simulink subsystem "Automotive_PowerTrain_AWDDifferential"  (R2024a)
settings: Solver=VariableStepAuto  StartTime=0.0  StopTime=10.0  RelTol=1e-3
libraries: autolibshareddiff x1
settings Model: Creator=USER  LastModifiedBy=USER

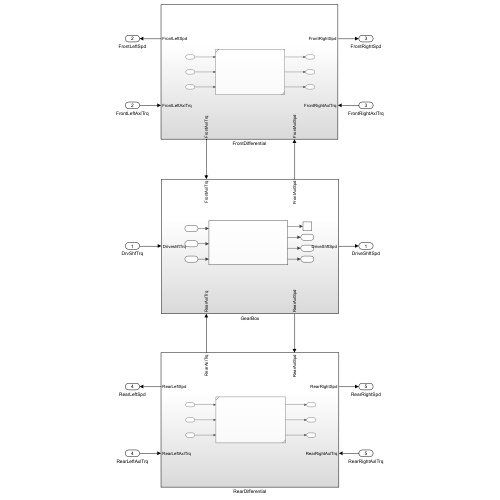
[thumbnail: Simulink's stored preview of the top-level diagram]
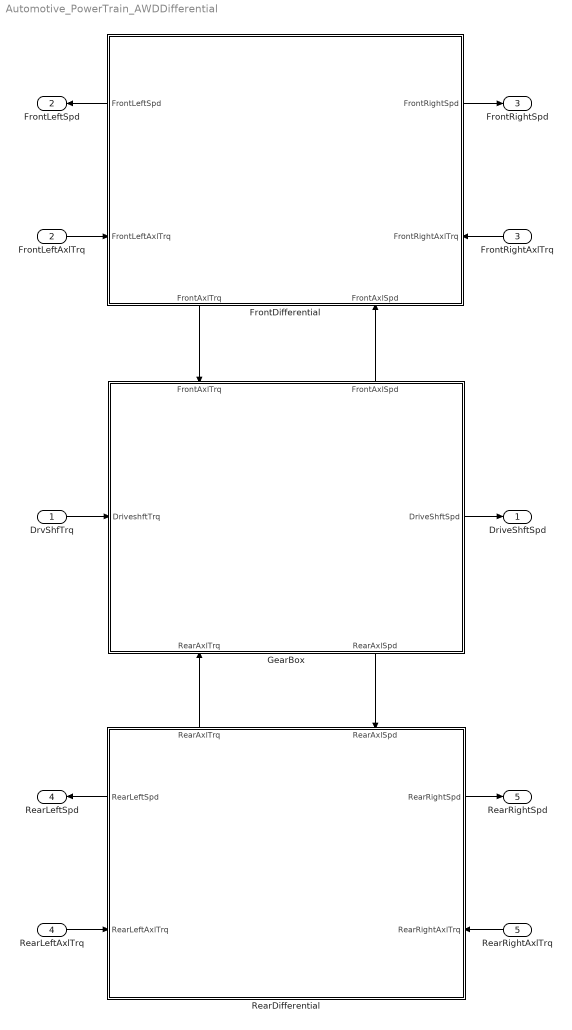
== system Automotive_PowerTrain_AWDDifferential ==
  DrvShfTrq : Inport
  FrontLeftAxlTrq : Inport  Port=2
  FrontRightAxlTrq : Inport  Port=3
  RearLeftAxlTrq : Inport  Port=4
  RearRightAxlTrq : Inport  Port=5
  FrontDifferential : Subsystem
      settings: PortSchema="{\"entries\":[{\"content\":{\"sides\":[{\"content\":{\"connectorIds\":[\"Out3\",\"In1\"]},\"type\":\"ConnectorPlacement.EquallySpacedRectSide\",\"uuid\":\"27f3256e-89ab-4368-8c78-2db926080991\"},{\"content\":{\"connectorIds\":[\"Out1\",\"In3\"],\"side\":\"RIGHT\"},\"type\":\"ConnectorPlacement.EquallySpacedRectSide\",\"uuid\":\"36e842ff-c4c6-4a20-acdc-cd70f8986d21\"},{\"content\":{\"side\":\"TOP\"},\"type\":\"ConnectorPlacement.EquallySpacedRectSide\",\"uuid\":\"2ccb2f9c-d9f3-4252-bb7a-d9380f21ab32\"},{\"content\":{\"connectorIds\":[\"Out2\",\"In2\"],\"side\":\"BOTTOM\"},\"type\":\"ConnectorPlacement.EquallySpacedRectSide\",\"uuid\":\"96e6a735-73c3-4e47-8511-c3716bbb9bc8\"}]},\"type\":\"ConnectorPlacement.EquallySpacedConnector\",\"uuid\":\"e81dde65-7a38-434f-9640-9946cbffd07c\"}],\"packageUris\":[\"http://schema.mathworks.com/mf0/Connector/R2020b\"],\"version\":\"1.0\"}"
  GearBox : Subsystem
      settings: PortSchema="{\"entries\":[{\"content\":{\"sides\":[{\"content\":{\"connectorIds\":[\"In1\"]},\"type\":\"ConnectorPlacement.EquallySpacedRectSide\",\"uuid\":\"27f3256e-89ab-4368-8c78-2db926080991\"},{\"content\":{\"connectorIds\":[\"Out1\"],\"side\":\"RIGHT\"},\"type\":\"ConnectorPlacement.EquallySpacedRectSide\",\"uuid\":\"36e842ff-c4c6-4a20-acdc-cd70f8986d21\"},{\"content\":{\"connectorIds\":[\"In2\",\"Out3\"],\"side\":\"TOP\"},\"type\":\"ConnectorPlacement.EquallySpacedRectSide\",\"uuid\":\"2ccb2f9c-d9f3-4252-bb7a-d9380f21ab32\"},{\"content\":{\"connectorIds\":[\"In3\",\"Out2\"],\"side\":\"BOTTOM\"},\"type\":\"ConnectorPlacement.EquallySpacedRectSide\",\"uuid\":\"f764fb99-6446-42c8-aaa9-dec82b0a64e1\"}]},\"type\":\"ConnectorPlacement.EquallySpacedConnector\",\"uuid\":\"e81dde65-7a38-434f-9640-9946cbffd07c\"}],\"packageUris\":[\"http://schema.mathworks.com/mf0/Connector/R2020b\"],\"version\":\"1.0\"}"
  RearDifferential : Subsystem
      settings: PortSchema="{\"entries\":[{\"content\":{\"sides\":[{\"content\":{\"connectorIds\":[\"Out3\",\"In1\"]},\"type\":\"ConnectorPlacement.EquallySpacedRectSide\",\"uuid\":\"27f3256e-89ab-4368-8c78-2db926080991\"},{\"content\":{\"connectorIds\":[\"Out1\",\"In3\"],\"side\":\"RIGHT\"},\"type\":\"ConnectorPlacement.EquallySpacedRectSide\",\"uuid\":\"36e842ff-c4c6-4a20-acdc-cd70f8986d21\"},{\"content\":{\"connectorIds\":[\"Out2\",\"In2\"],\"side\":\"TOP\"},\"type\":\"ConnectorPlacement.EquallySpacedRectSide\",\"uuid\":\"2ccb2f9c-d9f3-4252-bb7a-d9380f21ab32\"},{\"content\":{\"side\":\"BOTTOM\"},\"type\":\"ConnectorPlacement.EquallySpacedRectSide\",\"uuid\":\"96e6a735-73c3-4e47-8511-c3716bbb9bc8\"}]},\"type\":\"ConnectorPlacement.EquallySpacedConnector\",\"uuid\":\"e81dde65-7a38-434f-9640-9946cbffd07c\"}],\"packageUris\":[\"http://schema.mathworks.com/mf0/Connector/R2020b\"],\"version\":\"1.0\"}"
  DriveShftSpd : Outport
  FrontLeftSpd : Outport  Port=2
  FrontRightSpd : Outport  Port=3
  RearLeftSpd : Outport  Port=4
  RearRightSpd : Outport  Port=5
  wires:
  DrvShfTrq/1 -> GearBox/1(DriveshftTrq)
  GearBox/1(DriveShftSpd) -> DriveShftSpd/1
  FrontDifferential/2(FrontAxlTrq) -> GearBox/2(FrontAxlTrq)
  GearBox/3(FrontAxlSpd) -> FrontDifferential/2(FrontAxlSpd)
  RearDifferential/2(RearAxlTrq) -> GearBox/3(RearAxlTrq)
  GearBox/2(RearAxlSpd) -> RearDifferential/2(RearAxlSpd)
  FrontLeftAxlTrq/1 -> FrontDifferential/1(FrontLeftAxlTrq)
  FrontRightAxlTrq/1 -> FrontDifferential/3(FrontRightAxlTrq)
  RearLeftAxlTrq/1 -> RearDifferential/1(RearLeftAxlTrq)
  RearRightAxlTrq/1 -> RearDifferential/3(RearRightAxlTrq)
  FrontDifferential/3(FrontLeftSpd) -> FrontLeftSpd/1
  FrontDifferential/1(FrontRightSpd) -> FrontRightSpd/1
  RearDifferential/3(RearLeftSpd) -> RearLeftSpd/1
  RearDifferential/1(RearRightSpd) -> RearRightSpd/1

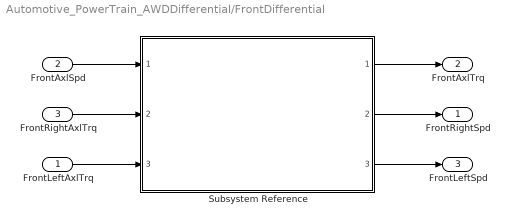
== system Automotive_PowerTrain_AWDDifferential/FrontDifferential ==
  FrontLeftAxlTrq : Inport
  FrontAxlSpd : Inport  Port=2
  FrontRightAxlTrq : Inport  Port=3
  Subsystem Reference : Subsystem  ReferencedSubsystem=Automotive_PowerTrain_OpenDifferential
  FrontRightSpd : Outport
  FrontAxlTrq : Outport  Port=2
  FrontLeftSpd : Outport  Port=3
  wires:
  FrontAxlSpd/1 -> Subsystem Reference/1
  FrontRightAxlTrq/1 -> Subsystem Reference/2
  FrontLeftAxlTrq/1 -> Subsystem Reference/3
  Subsystem Reference/1 -> FrontAxlTrq/1
  Subsystem Reference/3 -> FrontLeftSpd/1
  Subsystem Reference/2 -> FrontRightSpd/1

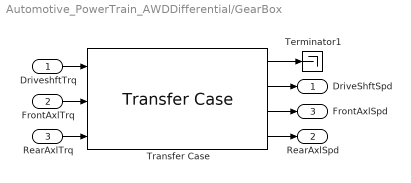
== system Automotive_PowerTrain_AWDDifferential/GearBox ==
  DriveshftTrq : Inport
  FrontAxlTrq : Inport  Port=2
  RearAxlTrq : Inport  Port=3
  Terminator1 : Terminator
  Transfer Case : autolibshareddiff/Transfer Case  DiffEffModelPopup=Constant  InterpMethod=Linear point-slope  extTamb=off  TrqSplitRatioMode=off  SpdLockMode=off  shaftSwitchMask=To the left of center-line  Ndiff=1  Jd=.1  bd=1e-3  Jw1=.1  bw1=1e-3  Jw2=.1  bw2=1e-3  omegaw1o=0  omegaw2o=0  eta=1  eta_tbl=reshape([0.64 0.76 0.8 0.81 0.83 0.84 0.84 0.56 0.73 0.78 0.8 0.83 0.84 0.84 0.54 0.71 0.77 0.8 0.82 0.84 0.84 0.53 0.71 0.77 0.8 0.83 0.84 0.84 0.51 0.71 0.77 0.8 0.83 0.84 0.85 0.52 0.7 0.77 0.8 0.83 0.84 0.85 0.51 0.71 0.76 0.79 0.83 0.84 0.85 0.5 0.69 0.76 0.79 0.82 0.84 0.85 0.45 0.68 0.75 0.78 0.82 0.84 0.85 0.43 0.67 0.74 0.78 0.81 0.83 0.84 0.38 0.63 0.71 0.75 0.8 0.82 0.83 0.81 0.86 0.88 0.89 0.89 0.89 0.9 0.77 0.85 0.87 0.88 0.89 0.9 0.9 0.72 0.82 0.86 0.87 0.88 0.89 0.9 0.68 0.8 0.84 0.86 0.88 0.89 0.89 0.67 0.8 0.84 0.86 0.88 0.89 0.9 0.67 0.8 0.84 0.86 0.88 0.89 0.9 0.65 0.8 0.84 0.86 0.88 0.89 0.9 0.64 0.79 0.83 0.86 0.88 0.89 0.9 0.63 0.78 0.83 0.86 0.88 0.89 0.9 0.59 0.76 0.82 0.85 0.87 0.89 0.9 0.53 0.73 0.8 0.83 0.86 0.88 0.89], 7, 11, 2)  Trq_bpts=[25, 50, 75, 100, 150, 200, 250]  omega_bpts=[52.4 78.5 105 131 157 183 209 262 314 419 524]  Temp_bpts=[290 358]  Tamb=297.15  maxAbsSpd=5e3  aMode=2  TrqSplitRatio=0.5  SpdLock=0
      settings: LibrarySourceBlock=vdynlib/Powertrain/Drivetrain/Final Drive Unit/Transfer Case
  DriveShftSpd : Outport  VectorParamsAs1DForOutWhenUnconnected=off
  RearAxlSpd : Outport  Port=2  VectorParamsAs1DForOutWhenUnconnected=off
  FrontAxlSpd : Outport  Port=3  VectorParamsAs1DForOutWhenUnconnected=off
  wires:
  DriveshftTrq/1 -> Transfer Case/1
  FrontAxlTrq/1 -> Transfer Case/2
  RearAxlTrq/1 -> Transfer Case/3
  Transfer Case/1 -> Terminator1/1
  Transfer Case/2 -> DriveShftSpd/1
  Transfer Case/3 -> FrontAxlSpd/1
  Transfer Case/4 -> RearAxlSpd/1

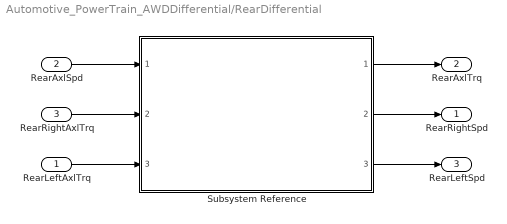
== system Automotive_PowerTrain_AWDDifferential/RearDifferential ==
  RearLeftAxlTrq : Inport
  RearAxlSpd : Inport  Port=2
  RearRightAxlTrq : Inport  Port=3
  Subsystem Reference : Subsystem  ReferencedSubsystem=Automotive_PowerTrain_LimitedSlipDifferential
  RearRightSpd : Outport
  RearAxlTrq : Outport  Port=2
  RearLeftSpd : Outport  Port=3
  wires:
  RearAxlSpd/1 -> Subsystem Reference/1
  RearRightAxlTrq/1 -> Subsystem Reference/2
  RearLeftAxlTrq/1 -> Subsystem Reference/3
  Subsystem Reference/1 -> RearAxlTrq/1
  Subsystem Reference/3 -> RearLeftSpd/1
  Subsystem Reference/2 -> RearRightSpd/1
